simulink model "radius"  (R2018b)
settings: Solver=VariableStepAuto  StartTime=0.0  StopTime=10.0  RelTol=1e-3
settings Model: Creator=Edoardo  LastModifiedBy=Edoardo

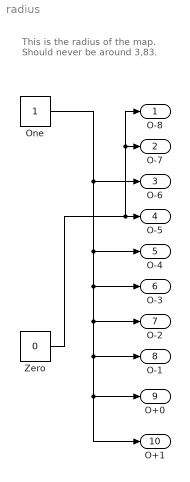
== system radius ==
  note: This is the radius of the map.
      | Should never be around 3,83.
  One : Constant  OutDataTypeStr=Inherit: Inherit via back propagation
  Zero : Constant  Value=0  OutDataTypeStr=Inherit: Inherit via back propagation
  "O-8 " : Outport  OutDataTypeStr=boolean
  O-7 : Outport  Port=2  OutDataTypeStr=boolean
  O-6 : Outport  Port=3  OutDataTypeStr=boolean
  "O-5 " : Outport  Port=4  OutDataTypeStr=boolean
  O-4 : Outport  Port=5  OutDataTypeStr=boolean
  O-3 : Outport  Port=6  OutDataTypeStr=boolean
  O-2 : Outport  Port=7  OutDataTypeStr=boolean
  O-1 : Outport  Port=8  OutDataTypeStr=boolean
  O+0 : Outport  Port=9  OutDataTypeStr=boolean
  O+1 : Outport  Port=10  OutDataTypeStr=boolean
  wires:
  One/1 -> O-4/1, O-3/1, O-2/1, O+0/1, O+1/1, O-1/1, O-6/1
  Zero/1 -> "O-8 "/1, O-7/1, "O-5 "/1
